simulink model "mStateflowDSMBasic"  (R2013b)
settings: Solver=FixedStepDiscrete  StartTime=0.0  StopTime=1  RelTol=1e-3
libraries: simulink x1
settings Model: Creator=hungdang  LastModifiedBy=hungdang
settings DataIOCC: SaveFormat=StructureWithTime
settings OptimizationCC: ActiveStateOutputEnumStorageType=Target Integer

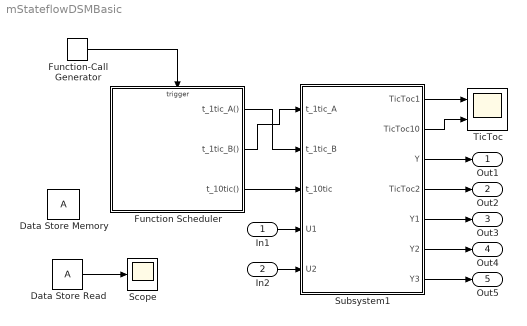
== system mStateflowDSMBasic ==
  In1 : Inport  OutDataTypeStr=double  PortDimensions=1  SampleTime=0.001
  In2 : Inport  Port=2  OutDataTypeStr=double  PortDimensions=1  SampleTime=0.001
  Data Store Memory : DataStoreMemory  ReadBeforeWriteMsg=warning  WriteAfterWriteMsg=warning  WriteAfterReadMsg=warning  OutDataTypeStr=int8
  Data Store Read : DataStoreRead
  Function Scheduler : Stateflow chart  TreatAsAtomicUnit=on
  Function-Call Generator : simulink/Ports & Subsystems/Function-Call Generator  sample_time=0.001  numberOfIterations=1
  Scope : Scope
  Subsystem1 : Subsystem
  TicToc : Scope  NumInputPorts=2
      settings: TimeRange=0.025  YMin=0~-1  YMax=1~1
  Out1 : Outport
  Out2 : Outport  Port=2
  Out3 : Outport  Port=3
  Out4 : Outport  Port=4
  Out5 : Outport  Port=5
  wires:
  Function-Call Generator/1 -> Function Scheduler/Trigger
  In1/1 -> Subsystem1/4(U1)
  In2/1 -> Subsystem1/5(U2)
  Subsystem1/3(Y) -> Out1/1
  Function Scheduler/3(t_10tic()) -> Subsystem1/3(t_10tic)
  Subsystem1/1(TicToc1) -> TicToc/1
  Subsystem1/2(TicToc10) -> TicToc/2
  Subsystem1/4(TicToc2) -> Out2/1
  Function Scheduler/1(t_1tic_A()) -> Subsystem1/2(t_1tic_B)
  Function Scheduler/2(t_1tic_B()) -> Subsystem1/1(t_1tic_A)
  Data Store Read/1 -> Scope/1
  Subsystem1/5(Y1) -> Out3/1
  Subsystem1/6(Y2) -> Out4/1
  Subsystem1/7(Y3) -> Out5/1

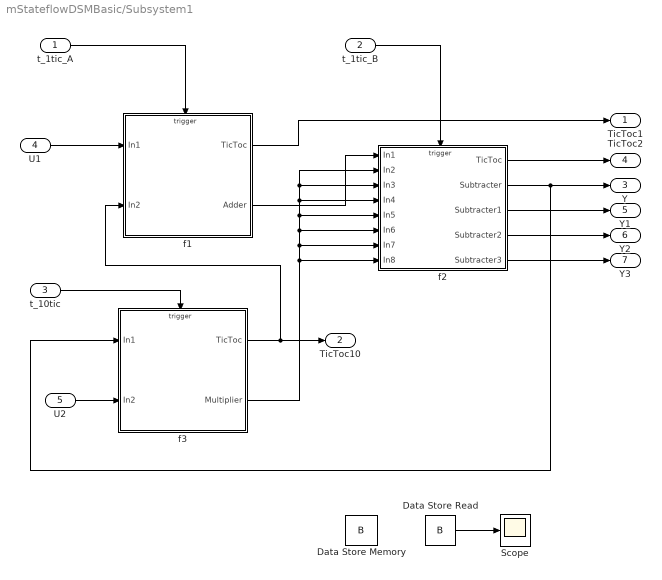
== system mStateflowDSMBasic/Subsystem1 ==
  t_1tic_A : Inport
  t_1tic_B : Inport  Port=2
  t_10tic : Inport  Port=3
  U1 : Inport  Port=4
  U2 : Inport  Port=5
  Data Store Memory : DataStoreMemory  DataStoreName=B  ReadBeforeWriteMsg=warning  WriteAfterWriteMsg=warning  WriteAfterReadMsg=warning  OutDataTypeStr=int8
  Data Store Read : DataStoreRead  DataStoreName=B
  Scope : Scope
      settings: SaveName=ScopeData2
  f1 : Subsystem  TreatAsAtomicUnit=on  RTWFcnName=foo
  f2 : Subsystem  TreatAsAtomicUnit=on  RTWFcnName=foo
  f3 : Subsystem  TreatAsAtomicUnit=on  RTWFcnName=foo
  TicToc1 : Outport
  TicToc10 : Outport  Port=2
  Y : Outport  Port=3
  TicToc2 : Outport  Port=4
  Y1 : Outport  Port=5
  Y2 : Outport  Port=6
  Y3 : Outport  Port=7
  wires:
  t_10tic/1 -> f3/Trigger
  U2/1 -> f3/2(In2)
  f2/2(Subtracter) -> f3/1(In1), Y/1
  f1/2(Adder) -> f2/1(In1)
  t_1tic_A/1 -> f1/Trigger
  f3/1(TicToc) -> f1/2(In2), TicToc10/1
  f2/1(TicToc) -> TicToc2/1
  f1/1(TicToc) -> TicToc1/1
  t_1tic_B/1 -> f2/Trigger
  U1/1 -> f1/1(In1)
  f2/3(Subtracter1) -> Y1/1
  f2/4(Subtracter2) -> Y2/1
  Data Store Read/1 -> Scope/1
  f3/2(Multiplier) -> f2/8(In8), f2/7(In7), f2/6(In6), f2/5(In5), f2/4(In4), f2/3(In3), f2/2(In2)
  f2/5(Subtracter3) -> Y3/1

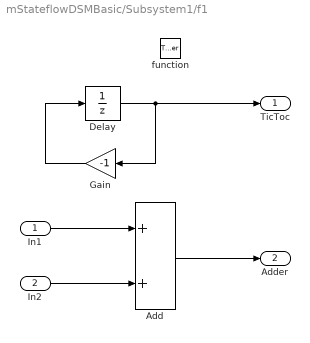
== system mStateflowDSMBasic/Subsystem1/f1 ==
  In1 : Inport
  In2 : Inport  Port=2
  function : TriggerPort  TriggerType=function-call
  Add : Sum
  Delay : UnitDelay  InitialCondition=1  SampleTime=-1
  Gain : Gain  Gain=-1  OutDataTypeStr=fixdt(1,8,0)
  TicToc : Outport  InitialOutput=0
  Adder : Outport  Port=2  InitialOutput=0
  wires:
  Add/1 -> Adder/1
  Gain/1 -> Delay/1
  Delay/1 -> TicToc/1, Gain/1
  In1/1 -> Add/1
  In2/1 -> Add/2

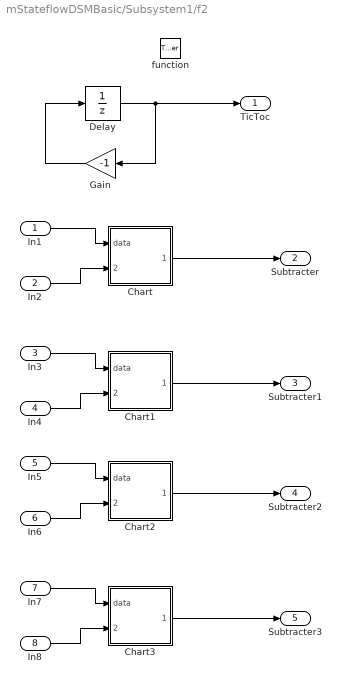
== system mStateflowDSMBasic/Subsystem1/f2 ==
  In1 : Inport
  In2 : Inport  Port=2
  In3 : Inport  Port=3
  In4 : Inport  Port=4
  In5 : Inport  Port=5
  In6 : Inport  Port=6
  In7 : Inport  Port=7
  In8 : Inport  Port=8
  function : TriggerPort  TriggerType=function-call
  Chart : Stateflow chart  TreatAsAtomicUnit=on
  Chart1 : Stateflow chart  TreatAsAtomicUnit=on
  Chart2 : Stateflow chart  TreatAsAtomicUnit=on
  Chart3 : Stateflow chart  TreatAsAtomicUnit=on
  Delay : UnitDelay  InitialCondition=1  SampleTime=-1
  Gain : Gain  Gain=-1  OutDataTypeStr=fixdt(1,8,0)
  TicToc : Outport  InitialOutput=0
  Subtracter : Outport  Port=2  InitialOutput=0
  Subtracter1 : Outport  Port=3  InitialOutput=0
  Subtracter2 : Outport  Port=4  InitialOutput=0
  Subtracter3 : Outport  Port=5  InitialOutput=0
  wires:
  In2/1 -> Chart/2(data1)
  In1/1 -> Chart/1(data)
  Delay/1 -> Gain/1, TicToc/1
  Gain/1 -> Delay/1
  Chart/1(data2) -> Subtracter/1
  In4/1 -> Chart1/2(data1)
  In3/1 -> Chart1/1(data)
  Chart1/1(data2) -> Subtracter1/1
  In6/1 -> Chart2/2(data1)
  In5/1 -> Chart2/1(data)
  Chart2/1(data2) -> Subtracter2/1
  In8/1 -> Chart3/2(data1)
  In7/1 -> Chart3/1(data)
  Chart3/1(data2) -> Subtracter3/1

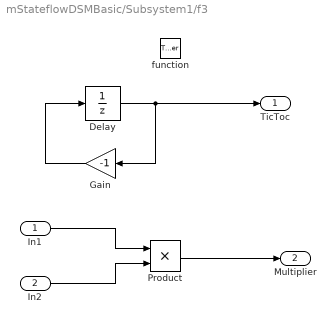
== system mStateflowDSMBasic/Subsystem1/f3 ==
  In1 : Inport
  In2 : Inport  Port=2
  function : TriggerPort  TriggerType=function-call
  Delay : UnitDelay  InitialCondition=1  SampleTime=-1
  Gain : Gain  Gain=-1  OutDataTypeStr=fixdt(1,8,0)
  Product : Product  Inputs=**  OutDataTypeStr=Inherit: Same as first input
  TicToc : Outport  InitialOutput=0
  Multiplier : Outport  Port=2  InitialOutput=0
  wires:
  In2/1 -> Product/2
  In1/1 -> Product/1
  Delay/1 -> Gain/1, TicToc/1
  Gain/1 -> Delay/1
  Product/1 -> Multiplier/1

== stateflow chart mStateflowDSMBasic/Function Scheduler ==
  settings: initializeOutput=1
  state OneTic [parallel]
    entry: t_1tic_B; t_1tic_A;
    on every(1,tic):
    t_1tic_B; t_1tic_A;
    settings: executionOrder=1
  state TenTic [parallel]
    entry: t_10tic;
    on every(10,tic): t_10tic;
    settings: executionOrder=2
  events: tic input FUNCTION_CALL_EVENT; t_1tic_A output FUNCTION_CALL_EVENT; t_1tic_B output FUNCTION_CALL_EVENT; t_10tic output FUNCTION_CALL_EVENT

== stateflow chart mStateflowDSMBasic/Subsystem1/f2/Chart ==
  (default) -> (junction 6) : {data2 = data + data1 + A;}
  data: data input; data1 input; data2 output double; A data_store_memory

== stateflow chart mStateflowDSMBasic/Subsystem1/f2/Chart1 ==
  (default) -> (junction 6) : {data2 = data + data1 + A;}
  data: data input; data1 input; data2 output double; A data_store_memory

== stateflow chart mStateflowDSMBasic/Subsystem1/f2/Chart2 ==
  (default) -> (junction 6) : {A = data + data1;}
  data: data input; data1 input; data2 output double; A data_store_memory

== stateflow chart mStateflowDSMBasic/Subsystem1/f2/Chart3 ==
  (default) -> (junction 6) : {B = data + data1;}
  data: data input; data1 input; data2 output double; B data_store_memory
